simulink model "vidu02"  (R2016a)
settings: Solver=VariableStepAuto  StartTime=0.0  StopTime=2000  RelTol=1e-3
settings Model: Creator=Lenovo  LastModifiedBy=Lenovo

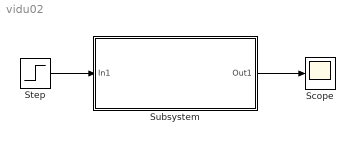
== system vidu02 ==
  Scope : Scope
  Step : Step  SampleTime=0
  Subsystem : Subsystem
  wires:
  Step/1 -> Subsystem/1(In1)
  Subsystem/1(Out1) -> Scope/1

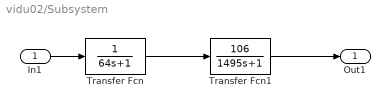
== system vidu02/Subsystem ==
  In1 : Inport
  Transfer Fcn : TransferFcn  Denominator=[64 1]
  Transfer Fcn1 : TransferFcn  Numerator=[106]  Denominator=[1495 1]
  Out1 : Outport
  wires:
  In1/1 -> Transfer Fcn/1
  Transfer Fcn1/1 -> Out1/1
  Transfer Fcn/1 -> Transfer Fcn1/1
